simulink model "SR_latch"  (R2020a)
settings: Solver=VariableStepAuto  StartTime=0.0  StopTime=inf  RelTol=1e-3
settings Model: Creator=F1  LastModifiedBy=F1

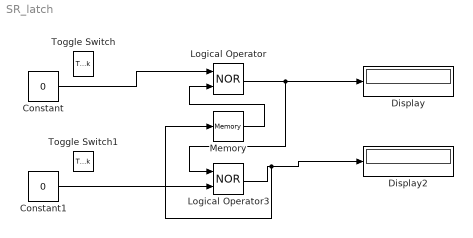
== system SR_latch ==
  Constant : Constant  Value=0
  Constant1 : Constant  Value=0
  Display : Display
  Display2 : Display
  Logical Operator : Logic  Operator=NOR  AllPortsSameDT=off  OutDataTypeStr=boolean
  Logical Operator3 : Logic  Operator=NOR  AllPortsSameDT=off  OutDataTypeStr=boolean
  Memory : Memory
  Toggle Switch : ToggleSwitchBlock
      settings: Values={{'Off', 'On'}, [0 1]}
  Toggle Switch1 : ToggleSwitchBlock
      settings: Values={{'Off', 'On'}, [0 1]}
  wires:
  Constant/1 -> Logical Operator/1
  Constant1/1 -> Logical Operator3/2
  Logical Operator3/1 -> Memory/1, Display2/1
  Logical Operator/1 -> Display/1, Logical Operator3/1
  Memory/1 -> Logical Operator/2
